simulink model "mlinear_SnookieConfiguration"  (R2017a)
settings: Solver=VariableStepAuto  StartTime=0.0  StopTime=10.0  RelTol=1e-3
undefined symbols (not defined in the file or in its folder): veh
libraries: sharedutil x6, sharedtransform x2, shared6dofsys x2
settings Model: Creator=yongyu  LastModifiedBy=yongyu

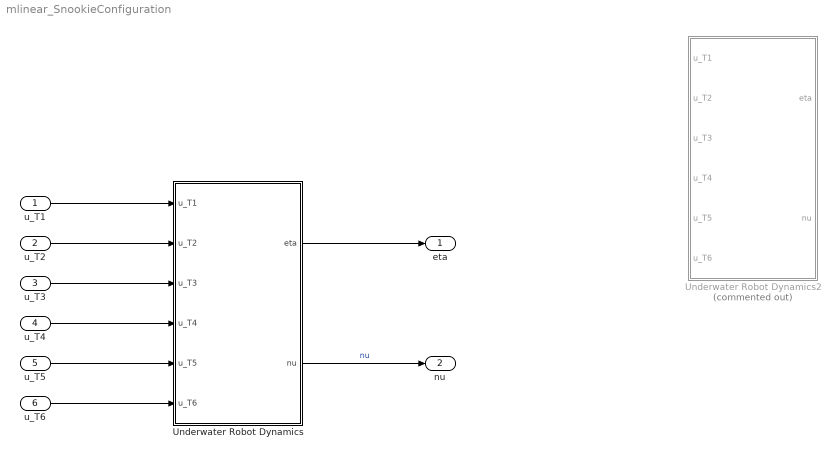
== system mlinear_SnookieConfiguration ==
  u_T1 : Inport
  u_T2 : Inport  Port=2
  u_T3 : Inport  Port=3
  u_T4 : Inport  Port=4
  u_T5 : Inport  Port=5
  u_T6 : Inport  Port=6
  Underwater Robot Dynamics : Subsystem
  Underwater Robot Dynamics2 : Subsystem  Commented=on
  eta : Outport
  nu : Outport  Port=2
  wires:
  u_T1/1 -> Underwater Robot Dynamics/1(u_T1)
  Underwater Robot Dynamics/1(eta) -> eta/1
  Underwater Robot Dynamics/2(nu) -> nu/1  "nu"
  u_T2/1 -> Underwater Robot Dynamics/2(u_T2)
  u_T3/1 -> Underwater Robot Dynamics/3(u_T3)
  u_T4/1 -> Underwater Robot Dynamics/4(u_T4)
  u_T5/1 -> Underwater Robot Dynamics/5(u_T5)
  u_T6/1 -> Underwater Robot Dynamics/6(u_T6)

== system mlinear_SnookieConfiguration/Underwater Robot Dynamics ==
  u_T1 : Inport
  u_T2 : Inport  Port=2
  u_T3 : Inport  Port=3
  u_T4 : Inport  Port=4
  u_T5 : Inport  Port=5
  u_T6 : Inport  Port=6
  ForceMomentTransfer : Subsystem
  Mux : Mux  Inputs=2
  Mux1 : Mux  Inputs=2
  Position Integrator(x,y,z) : Integrator
  Subsystem : Subsystem
  Transpose : Math  Operator=transpose  SaturateOnIntegerOverflow=on
  "Underwater Robot Dynamics " : Subsystem
  "transform to inertial world frame {i}" : Subsystem
  eta : Outport
  nu : Outport  Port=2
  wires:
  Transpose/1 -> "transform to inertial world frame {i}"/2(linear velocity transformation matrix)
  Mux1/1 -> nu/1  "nu"
  Mux/1 -> eta/1
  "transform to inertial world frame {i}"/1(Ve) -> Position Integrator(x,y,z)/1
  Position Integrator(x,y,z)/1 -> Mux/1
  "Underwater Robot Dynamics "/2(w_ib) -> Subsystem/1("p q r "), Mux1/2
  "Underwater Robot Dynamics "/1(v) -> Mux1/1, "transform to inertial world frame {i}"/1(v)
  Subsystem/1(DCM) -> Transpose/1
  Subsystem/2(Euler) -> Mux/2
  u_T1/1 -> ForceMomentTransfer/1(u_T1)
  u_T2/1 -> ForceMomentTransfer/2(u_T2)
  u_T3/1 -> ForceMomentTransfer/3(u_T3)
  u_T4/1 -> ForceMomentTransfer/4(u_T4)
  u_T5/1 -> ForceMomentTransfer/5(u_T5)
  u_T6/1 -> ForceMomentTransfer/6(u_T6)
  ForceMomentTransfer/1(tau_b) -> "Underwater Robot Dynamics "/1(tau_b)

== system mlinear_SnookieConfiguration/Underwater Robot Dynamics2 ==
  u_T1 : Inport
  u_T2 : Inport  Port=2
  u_T3 : Inport  Port=3
  u_T4 : Inport  Port=4
  u_T5 : Inport  Port=5
  u_T6 : Inport  Port=6
  ForceMomentTransfer : Subsystem
  Mux : Mux  Inputs=2
  Mux1 : Mux  Inputs=2
  Position Integrator(x,y,z) : Integrator
  Subsystem : Subsystem
  Transpose : Math  Operator=transpose  SaturateOnIntegerOverflow=on
  "Underwater Robot Dynamics " : Subsystem
  "transform to inertial world frame {i}" : Subsystem
  eta : Outport
  nu : Outport  Port=2
  wires:
  Transpose/1 -> "transform to inertial world frame {i}"/2(linear velocity transformation matrix)
  Mux1/1 -> nu/1  "nu"
  Mux/1 -> eta/1
  "transform to inertial world frame {i}"/1(Ve) -> Position Integrator(x,y,z)/1
  Position Integrator(x,y,z)/1 -> Mux/1
  "Underwater Robot Dynamics "/2(w_ib) -> Subsystem/1("p q r "), Mux1/2
  "Underwater Robot Dynamics "/1(v) -> Mux1/1, "transform to inertial world frame {i}"/1(v)
  Subsystem/1(DCM) -> Transpose/1
  Subsystem/2(Euler) -> Mux/2
  u_T1/1 -> ForceMomentTransfer/1(u_T1)
  u_T2/1 -> ForceMomentTransfer/2(u_T2)
  u_T3/1 -> ForceMomentTransfer/3(u_T3)
  u_T4/1 -> ForceMomentTransfer/4(u_T4)
  u_T5/1 -> ForceMomentTransfer/5(u_T5)
  u_T6/1 -> ForceMomentTransfer/6(u_T6)
  ForceMomentTransfer/1(tau_b) -> "Underwater Robot Dynamics "/1(tau_b)

== system mlinear_SnookieConfiguration/Underwater Robot Dynamics/ForceMomentTransfer ==
  u_T1 : Inport
  u_T2 : Inport  Port=2
  u_T3 : Inport  Port=3
  u_T4 : Inport  Port=4
  u_T5 : Inport  Port=5
  u_T6 : Inport  Port=6
  Mux : Mux  Inputs=2
  Total Force : Subsystem
  Total Moment : Subsystem
  tau_b : Outport
  wires:
  u_T1/1 -> Total Moment/1(u_T1), Total Force/1(u_T1)
  u_T2/1 -> Total Moment/2(u_T2), Total Force/2(u_T2)
  u_T3/1 -> Total Force/3(u_T3), Total Moment/3(u_T3)
  u_T4/1 -> Total Force/4(u_T4), Total Moment/4(u_T4)
  u_T5/1 -> Total Force/5(u_T5), Total Moment/5(u_T5)
  u_T6/1 -> Total Force/6(u_T6), Total Moment/6(u_T6)
  Total Force/1(F_T) -> Mux/1
  Total Moment/1(m_T) -> Mux/2
  Mux/1 -> tau_b/1

== system mlinear_SnookieConfiguration/Underwater Robot Dynamics/Subsystem ==
  "p q r " : Inport
  Rotation Angles to Direction Cosine Matrix : sharedtransform/Rotation Angles to Direction Cosine Matrix  rotationOrder=ZYX
  Selector : Selector  InputPortWidth=3  IndexOptions=Index vector (dialog)  Indices=[3 2 1]  OutputSizes=1
  phi theta psi : Integrator
  phidot thetadot psidot : shared6dofsys/DCM & Euler Angles (Euler)/phidot thetadot psidot
  DCM : Outport
  Euler : Outport  Port=2
  wires:
  Selector/1 -> Rotation Angles to Direction Cosine Matrix/1
  "p q r "/1 -> phidot thetadot psidot/1
  phi theta psi/1 -> Euler/1, Selector/1, phidot thetadot psidot/2
  phidot thetadot psidot/1 -> phi theta psi/1
  Rotation Angles to Direction Cosine Matrix/1 -> DCM/1

== system mlinear_SnookieConfiguration/Underwater Robot Dynamics/Underwater Robot Dynamics  ==
  tau_b : Inport
  6DOF Coriolis forces : Subsystem
  M_A : Constant  Value=veh.Ma
  M_RB : Constant  Value=veh.Mrb
  Product : Product  Inputs=/*  Multiplication=Matrix(*)  SaturateOnIntegerOverflow=on  OutDataTypeStr=Inherit: Same as first input
  Scope : Scope
  Selector1 : Selector  InputPortWidth=6  IndexOptions=Index vector (dialog)  Indices=[1 2 3]  OutputSizes=1
  Selector2 : Selector  InputPortWidth=6  IndexOptions=Index vector (dialog)  Indices=[4 5 6]  OutputSizes=1
  Sum : Sum  Inputs=|+-
  Sum2 : Sum  SaturateOnIntegerOverflow=on
  Velocity Integrator : Integrator
  v : Outport
  w_ib : Outport  Port=2
  wires:
  M_RB/1 -> Sum2/1
  M_A/1 -> Sum2/2
  Sum2/1 -> Product/1, 6DOF Coriolis forces/1(M)  "M"
  Selector2/1 -> w_ib/1  "w_nb"
  Product/1 -> Velocity Integrator/1  "(d/dt)nu"
  6DOF Coriolis forces/1(C(nu)nu) -> Sum/2, Scope/1
  Sum/1 -> Product/2
  Selector1/1 -> v/1  "v"
  Velocity Integrator/1 -> 6DOF Coriolis forces/2(nu), Selector2/1, Selector1/1  "nu"
  tau_b/1 -> Sum/1

== system mlinear_SnookieConfiguration/Underwater Robot Dynamics/transform to inertial world frame {i} ==
  v : Inport
  linear velocity transformation matrix : Inport  Port=2
  Product : Product  Multiplication=Matrix(*)  SaturateOnIntegerOverflow=on  InputSameDT=on  OutDataTypeStr=Inherit: Same as first input
  Reshape1 : Reshape  OutputDimensionality=Column vector (2-D)
  Reshape2 : Reshape
  Ve : Outport
  wires:
  Product/1 -> Reshape2/1
  Reshape1/1 -> Product/2
  v/1 -> Reshape1/1
  Reshape2/1 -> Ve/1
  linear velocity transformation matrix/1 -> Product/1

== system mlinear_SnookieConfiguration/Underwater Robot Dynamics2/ForceMomentTransfer ==
  u_T1 : Inport
  u_T2 : Inport  Port=2
  u_T3 : Inport  Port=3
  u_T4 : Inport  Port=4
  u_T5 : Inport  Port=5
  u_T6 : Inport  Port=6
  Mux : Mux  Inputs=2
  Total Force : Subsystem
  Total Moment : Subsystem
  tau_b : Outport
  wires:
  u_T1/1 -> Total Moment/1(u_T1), Total Force/1(u_T1)
  u_T2/1 -> Total Moment/2(u_T2), Total Force/2(u_T2)
  u_T3/1 -> Total Force/3(u_T3), Total Moment/3(u_T3)
  u_T4/1 -> Total Force/4(u_T4), Total Moment/4(u_T4)
  u_T5/1 -> Total Force/5(u_T5), Total Moment/5(u_T5)
  u_T6/1 -> Total Force/6(u_T6), Total Moment/6(u_T6)
  Total Force/1(F_T) -> Mux/1
  Total Moment/1(m_T) -> Mux/2
  Mux/1 -> tau_b/1

== system mlinear_SnookieConfiguration/Underwater Robot Dynamics2/Subsystem ==
  "p q r " : Inport
  Rotation Angles to Direction Cosine Matrix : sharedtransform/Rotation Angles to Direction Cosine Matrix  rotationOrder=ZYX
  Selector : Selector  InputPortWidth=3  IndexOptions=Index vector (dialog)  Indices=[3 2 1]  OutputSizes=1
  phi theta psi : Integrator
  phidot thetadot psidot : shared6dofsys/DCM & Euler Angles (Euler)/phidot thetadot psidot
  DCM : Outport
  Euler : Outport  Port=2
  wires:
  Selector/1 -> Rotation Angles to Direction Cosine Matrix/1
  "p q r "/1 -> phidot thetadot psidot/1
  phi theta psi/1 -> Euler/1, Selector/1, phidot thetadot psidot/2
  phidot thetadot psidot/1 -> phi theta psi/1
  Rotation Angles to Direction Cosine Matrix/1 -> DCM/1

== system mlinear_SnookieConfiguration/Underwater Robot Dynamics2/Underwater Robot Dynamics  ==
  tau_b : Inport
  6DOF Coriolis forces : Subsystem
  M_A : Constant  Value=veh.Ma
  M_RB : Constant  Value=veh.Mrb
  Product : Product  Inputs=/*  Multiplication=Matrix(*)  SaturateOnIntegerOverflow=on  OutDataTypeStr=Inherit: Same as first input
  Scope : Scope
  Selector1 : Selector  InputPortWidth=6  IndexOptions=Index vector (dialog)  Indices=[1 2 3]  OutputSizes=1
  Selector2 : Selector  InputPortWidth=6  IndexOptions=Index vector (dialog)  Indices=[4 5 6]  OutputSizes=1
  Sum : Sum  Inputs=|+-
  Sum2 : Sum  SaturateOnIntegerOverflow=on
  Velocity Integrator : Integrator
  v : Outport
  w_ib : Outport  Port=2
  wires:
  M_RB/1 -> Sum2/1
  M_A/1 -> Sum2/2
  Sum2/1 -> Product/1, 6DOF Coriolis forces/1(M)  "M"
  Selector2/1 -> w_ib/1  "w_nb"
  Product/1 -> Velocity Integrator/1  "(d/dt)nu"
  6DOF Coriolis forces/1(C(nu)nu) -> Sum/2, Scope/1
  Sum/1 -> Product/2
  Selector1/1 -> v/1  "v"
  Velocity Integrator/1 -> 6DOF Coriolis forces/2(nu), Selector2/1, Selector1/1  "nu"
  tau_b/1 -> Sum/1

== system mlinear_SnookieConfiguration/Underwater Robot Dynamics2/transform to inertial world frame {i} ==
  v : Inport
  linear velocity transformation matrix : Inport  Port=2
  Product : Product  Multiplication=Matrix(*)  SaturateOnIntegerOverflow=on  InputSameDT=on  OutDataTypeStr=Inherit: Same as first input
  Reshape1 : Reshape  OutputDimensionality=Column vector (2-D)
  Reshape2 : Reshape
  Ve : Outport
  wires:
  Product/1 -> Reshape2/1
  Reshape1/1 -> Product/2
  v/1 -> Reshape1/1
  Reshape2/1 -> Ve/1
  linear velocity transformation matrix/1 -> Product/1

== system mlinear_SnookieConfiguration/Underwater Robot Dynamics/ForceMomentTransfer/Total Force ==
  u_T1 : Inport
  u_T2 : Inport  Port=2
  u_T3 : Inport  Port=3
  u_T4 : Inport  Port=4
  u_T5 : Inport  Port=5
  u_T6 : Inport  Port=6
  Add : Sum  Inputs=++++++
  Gain : Gain  Gain=veh.d_T1
  Gain1 : Gain  Gain=veh.d_T2
  Gain2 : Gain  Gain=veh.d_T3
  Gain3 : Gain  Gain=veh.d_T4
  Gain4 : Gain  Gain=veh.d_T5
  Gain5 : Gain  Gain=veh.d_T6
  F_T : Outport
  wires:
  Add/1 -> F_T/1
  u_T1/1 -> Gain/1
  Gain/1 -> Add/1
  Gain1/1 -> Add/2
  Gain2/1 -> Add/3
  u_T2/1 -> Gain1/1
  u_T3/1 -> Gain2/1
  Gain3/1 -> Add/4
  u_T4/1 -> Gain3/1
  u_T5/1 -> Gain4/1
  Gain4/1 -> Add/5
  u_T6/1 -> Gain5/1
  Gain5/1 -> Add/6

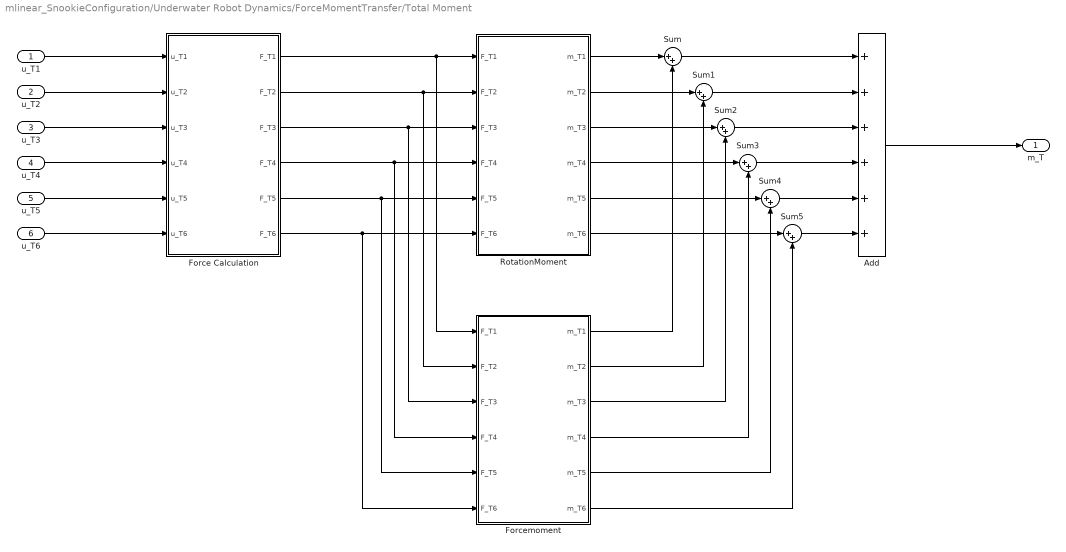
== system mlinear_SnookieConfiguration/Underwater Robot Dynamics/ForceMomentTransfer/Total Moment ==
  u_T1 : Inport
  u_T2 : Inport  Port=2
  u_T3 : Inport  Port=3
  u_T4 : Inport  Port=4
  u_T5 : Inport  Port=5
  u_T6 : Inport  Port=6
  Add : Sum  Inputs=++++++
  "Force Calculation " : Subsystem
  Forcemoment : Subsystem
  RotationMoment : Subsystem
  Sum{,1..5} (6 alike) : Sum  Inputs=|++
  m_T : Outport
  wires:
  Add/1 -> m_T/1
  "Force Calculation "/1(F_T1) -> Forcemoment/1(F_T1), RotationMoment/1(F_T1)
  "Force Calculation "/2(F_T2) -> Forcemoment/2(F_T2), RotationMoment/2(F_T2)
  "Force Calculation "/3(F_T3) -> Forcemoment/3(F_T3), RotationMoment/3(F_T3)
  "Force Calculation "/5(F_T5) -> Forcemoment/5(F_T5), RotationMoment/5(F_T5)
  "Force Calculation "/4(F_T4) -> Forcemoment/4(F_T4), RotationMoment/4(F_T4)
  "Force Calculation "/6(F_T6) -> Forcemoment/6(F_T6), RotationMoment/6(F_T6)
  RotationMoment/1(m_T1) -> Sum/1
  Forcemoment/1(m_T1) -> Sum/2
  RotationMoment/2(m_T2) -> Sum1/1
  Forcemoment/2(m_T2) -> Sum1/2
  RotationMoment/3(m_T3) -> Sum2/1
  Forcemoment/3(m_T3) -> Sum2/2
  RotationMoment/4(m_T4) -> Sum3/1
  Forcemoment/4(m_T4) -> Sum3/2
  RotationMoment/5(m_T5) -> Sum4/1
  Forcemoment/5(m_T5) -> Sum4/2
  RotationMoment/6(m_T6) -> Sum5/1
  Forcemoment/6(m_T6) -> Sum5/2
  Sum/1 -> Add/1
  Sum1/1 -> Add/2
  Sum2/1 -> Add/3
  Sum3/1 -> Add/4
  Sum4/1 -> Add/5
  Sum5/1 -> Add/6
  u_T1/1 -> "Force Calculation "/1(u_T1)
  u_T2/1 -> "Force Calculation "/2(u_T2)
  u_T3/1 -> "Force Calculation "/3(u_T3)
  u_T4/1 -> "Force Calculation "/4(u_T4)
  u_T5/1 -> "Force Calculation "/5(u_T5)
  u_T6/1 -> "Force Calculation "/6(u_T6)

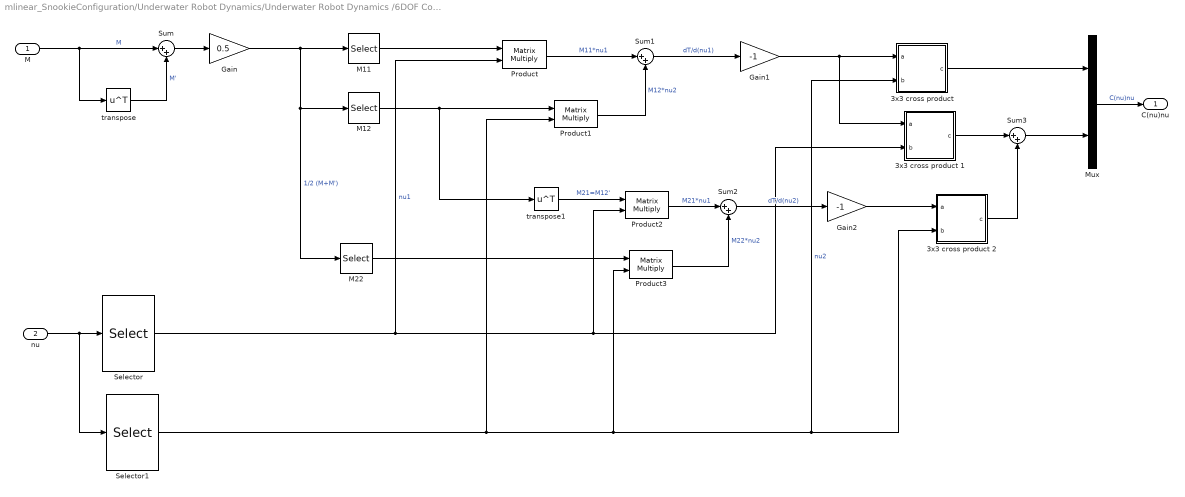
== system mlinear_SnookieConfiguration/Underwater Robot Dynamics/Underwater Robot Dynamics /6DOF Coriolis forces ==
  M : Inport
  nu : Inport  Port=2
  3x3 cross product : Subsystem
  3x3 cross product 1 : Subsystem
  3x3 cross product 2 : Subsystem
  Gain : Gain  Gain=0.5  SaturateOnIntegerOverflow=on  OutDataTypeStr=Inherit: Same as input  ParamDataTypeStr=Inherit: Same as input
  Gain1 : Gain  Gain=-1  SaturateOnIntegerOverflow=on  OutDataTypeStr=Inherit: Same as input  ParamDataTypeStr=Inherit: Same as input
  Gain2 : Gain  Gain=-1  SaturateOnIntegerOverflow=on  OutDataTypeStr=Inherit: Same as input  ParamDataTypeStr=Inherit: Same as input
  M11 : Selector  NumberOfDimensions=2  InputPortWidth=3  IndexOptions=Index vector (dialog),Index vector (dialog)  Indices=[1 2 3],[1 2 3]  OutputSizes=1
  M12 : Selector  NumberOfDimensions=2  InputPortWidth=3  IndexOptions=Index vector (dialog),Index vector (dialog)  Indices=[1 2 3],[4 5 6]  OutputSizes=1
  M22 : Selector  NumberOfDimensions=2  InputPortWidth=3  IndexOptions=Index vector (dialog),Index vector (dialog)  Indices=[4 5 6],[4 5 6]  OutputSizes=1
  Mux : Mux  Inputs=2
  Product{,1..3} (4 alike) : Product  Multiplication=Matrix(*)  SaturateOnIntegerOverflow=on  OutDataTypeStr=Inherit: Same as first input
  Selector : Selector  InputPortWidth=6  IndexOptions=Index vector (dialog)  Indices=[1 2 3]  OutputSizes=1
  Selector1 : Selector  InputPortWidth=6  IndexOptions=Index vector (dialog)  Indices=[4 5 6]  OutputSizes=1
  Sum{,1..3} (4 alike) : Sum  Inputs=|++  SaturateOnIntegerOverflow=on
  transpose : Math  Operator=transpose  SaturateOnIntegerOverflow=on
  transpose1 : Math  Operator=transpose  SaturateOnIntegerOverflow=on
  C(nu)nu : Outport
  wires:
  transpose/1 -> Sum/2  "M'"
  Sum/1 -> Gain/1
  Gain/1 -> M22/1, M12/1, M11/1  "1/2 (M+M')"
  Selector/1 -> Product2/2, 3x3 cross product 1/2(b), Product/2  "nu1"
  Selector1/1 -> 3x3 cross product/2(b), 3x3 cross product 2/2(b), Product3/2, Product1/2  "nu2"
  M11/1 -> Product/1
  Product/1 -> Sum1/1  "M11*nu1"
  M12/1 -> transpose1/1, Product1/1
  Product1/1 -> Sum1/2  "M12*nu2"
  Sum1/1 -> Gain1/1  "dT/d(nu1)"
  transpose1/1 -> Product2/1  "M21=M12'"
  Product2/1 -> Sum2/1  "M21*nu1"
  M22/1 -> Product3/1
  Product3/1 -> Sum2/2  "M22*nu2"
  Sum2/1 -> Gain2/1  "dT/d(nu2)"
  Gain1/1 -> 3x3 cross product/1(a), 3x3 cross product 1/1(a)
  3x3 cross product/1(c) -> Mux/1
  Gain2/1 -> 3x3 cross product 2/1(a)
  3x3 cross product 1/1(c) -> Sum3/1
  3x3 cross product 2/1(c) -> Sum3/2
  Sum3/1 -> Mux/2
  Mux/1 -> C(nu)nu/1  "C(nu)nu"
  nu/1 -> Selector/1, Selector1/1
  M/1 -> transpose/1, Sum/1  "M"

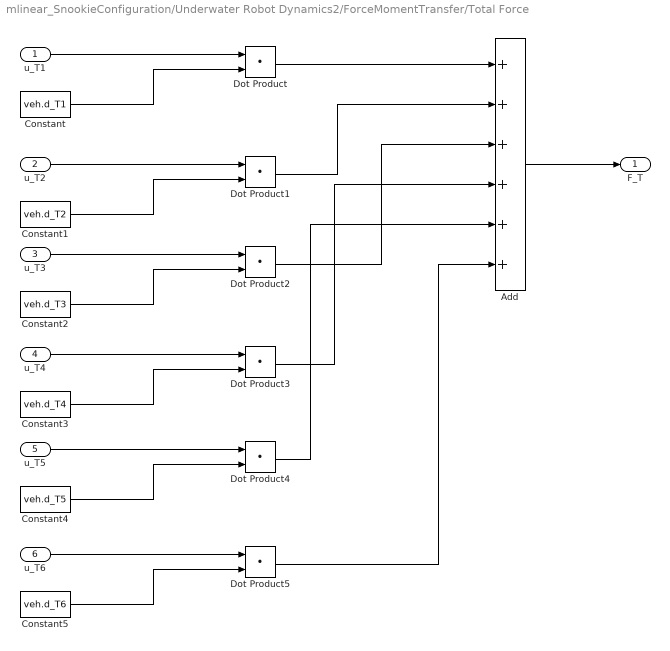
== system mlinear_SnookieConfiguration/Underwater Robot Dynamics2/ForceMomentTransfer/Total Force ==
  u_T1 : Inport
  u_T2 : Inport  Port=2
  u_T3 : Inport  Port=3
  u_T4 : Inport  Port=4
  u_T5 : Inport  Port=5
  u_T6 : Inport  Port=6
  Add : Sum  Inputs=++++++
  Constant : Constant  Value=veh.d_T1
  Constant1 : Constant  Value=veh.d_T2
  Constant2 : Constant  Value=veh.d_T3
  Constant3 : Constant  Value=veh.d_T4
  Constant4 : Constant  Value=veh.d_T5
  Constant5 : Constant  Value=veh.d_T6
  Dot Product{,1..5} (6 alike) : DotProduct  InputSameDT=on  OutDataTypeStr=Inherit: Inherit via internal rule
  F_T : Outport
  wires:
  Add/1 -> F_T/1
  u_T1/1 -> Dot Product/1
  Constant/1 -> Dot Product/2
  Dot Product/1 -> Add/1
  Constant1/1 -> Dot Product1/2
  u_T2/1 -> Dot Product1/1
  Dot Product1/1 -> Add/2
  u_T3/1 -> Dot Product2/1
  Constant2/1 -> Dot Product2/2
  Dot Product2/1 -> Add/3
  u_T4/1 -> Dot Product3/1
  Constant3/1 -> Dot Product3/2
  Dot Product3/1 -> Add/4
  u_T5/1 -> Dot Product4/1
  Constant4/1 -> Dot Product4/2
  u_T6/1 -> Dot Product5/1
  Constant5/1 -> Dot Product5/2
  Dot Product4/1 -> Add/5
  Dot Product5/1 -> Add/6

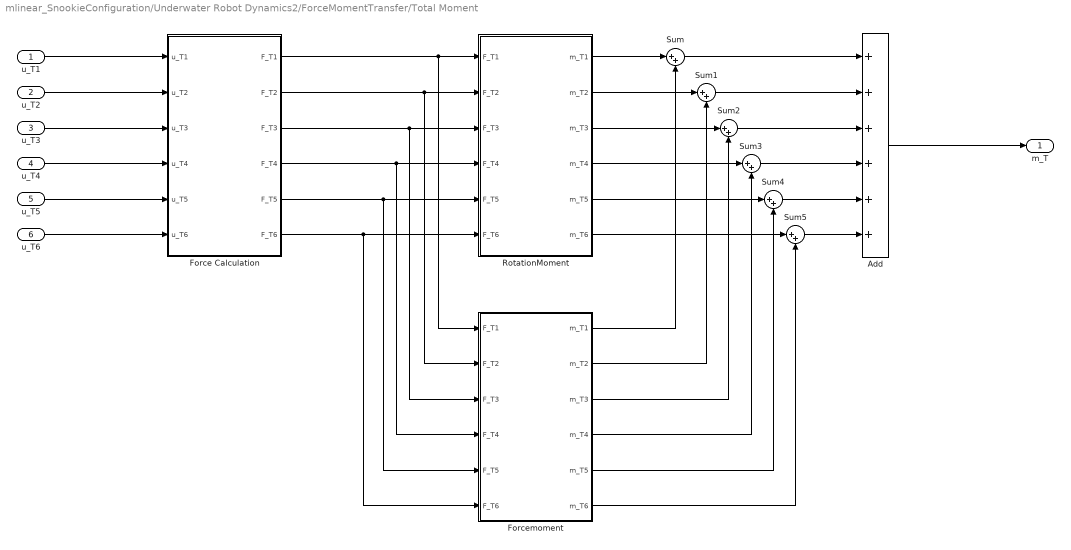
== system mlinear_SnookieConfiguration/Underwater Robot Dynamics2/ForceMomentTransfer/Total Moment ==
  u_T1 : Inport
  u_T2 : Inport  Port=2
  u_T3 : Inport  Port=3
  u_T4 : Inport  Port=4
  u_T5 : Inport  Port=5
  u_T6 : Inport  Port=6
  Add : Sum  Inputs=++++++
  "Force Calculation " : Subsystem
  Forcemoment : Subsystem
  RotationMoment : Subsystem
  Sum{,1..5} (6 alike) : Sum  Inputs=|++
  m_T : Outport
  wires:
  Add/1 -> m_T/1
  u_T1/1 -> "Force Calculation "/1(u_T1)
  u_T3/1 -> "Force Calculation "/3(u_T3)
  u_T4/1 -> "Force Calculation "/4(u_T4)
  u_T2/1 -> "Force Calculation "/2(u_T2)
  u_T5/1 -> "Force Calculation "/5(u_T5)
  u_T6/1 -> "Force Calculation "/6(u_T6)
  "Force Calculation "/1(F_T1) -> Forcemoment/1(F_T1), RotationMoment/1(F_T1)
  "Force Calculation "/2(F_T2) -> Forcemoment/2(F_T2), RotationMoment/2(F_T2)
  "Force Calculation "/3(F_T3) -> Forcemoment/3(F_T3), RotationMoment/3(F_T3)
  "Force Calculation "/5(F_T5) -> Forcemoment/5(F_T5), RotationMoment/5(F_T5)
  "Force Calculation "/4(F_T4) -> Forcemoment/4(F_T4), RotationMoment/4(F_T4)
  "Force Calculation "/6(F_T6) -> Forcemoment/6(F_T6), RotationMoment/6(F_T6)
  RotationMoment/1(m_T1) -> Sum/1
  Forcemoment/1(m_T1) -> Sum/2
  RotationMoment/2(m_T2) -> Sum1/1
  Forcemoment/2(m_T2) -> Sum1/2
  RotationMoment/3(m_T3) -> Sum2/1
  Forcemoment/3(m_T3) -> Sum2/2
  RotationMoment/4(m_T4) -> Sum3/1
  Forcemoment/4(m_T4) -> Sum3/2
  RotationMoment/5(m_T5) -> Sum4/1
  Forcemoment/5(m_T5) -> Sum4/2
  RotationMoment/6(m_T6) -> Sum5/1
  Forcemoment/6(m_T6) -> Sum5/2
  Sum/1 -> Add/1
  Sum1/1 -> Add/2
  Sum2/1 -> Add/3
  Sum3/1 -> Add/4
  Sum4/1 -> Add/5
  Sum5/1 -> Add/6

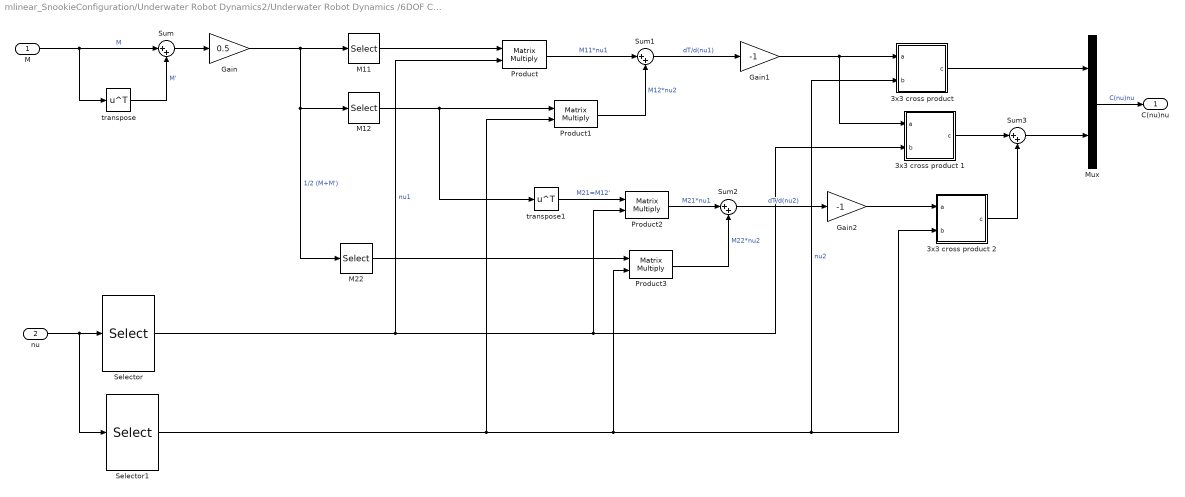
== system mlinear_SnookieConfiguration/Underwater Robot Dynamics2/Underwater Robot Dynamics /6DOF Coriolis forces ==
  M : Inport
  nu : Inport  Port=2
  3x3 cross product : Subsystem
  3x3 cross product 1 : Subsystem
  3x3 cross product 2 : Subsystem
  Gain : Gain  Gain=0.5  SaturateOnIntegerOverflow=on  OutDataTypeStr=Inherit: Same as input  ParamDataTypeStr=Inherit: Same as input
  Gain1 : Gain  Gain=-1  SaturateOnIntegerOverflow=on  OutDataTypeStr=Inherit: Same as input  ParamDataTypeStr=Inherit: Same as input
  Gain2 : Gain  Gain=-1  SaturateOnIntegerOverflow=on  OutDataTypeStr=Inherit: Same as input  ParamDataTypeStr=Inherit: Same as input
  M11 : Selector  NumberOfDimensions=2  InputPortWidth=3  IndexOptions=Index vector (dialog),Index vector (dialog)  Indices=[1 2 3],[1 2 3]  OutputSizes=1
  M12 : Selector  NumberOfDimensions=2  InputPortWidth=3  IndexOptions=Index vector (dialog),Index vector (dialog)  Indices=[1 2 3],[4 5 6]  OutputSizes=1
  M22 : Selector  NumberOfDimensions=2  InputPortWidth=3  IndexOptions=Index vector (dialog),Index vector (dialog)  Indices=[4 5 6],[4 5 6]  OutputSizes=1
  Mux : Mux  Inputs=2
  Product{,1..3} (4 alike) : Product  Multiplication=Matrix(*)  SaturateOnIntegerOverflow=on  OutDataTypeStr=Inherit: Same as first input
  Selector : Selector  InputPortWidth=6  IndexOptions=Index vector (dialog)  Indices=[1 2 3]  OutputSizes=1
  Selector1 : Selector  InputPortWidth=6  IndexOptions=Index vector (dialog)  Indices=[4 5 6]  OutputSizes=1
  Sum{,1..3} (4 alike) : Sum  Inputs=|++  SaturateOnIntegerOverflow=on
  transpose : Math  Operator=transpose  SaturateOnIntegerOverflow=on
  transpose1 : Math  Operator=transpose  SaturateOnIntegerOverflow=on
  C(nu)nu : Outport
  wires:
  transpose/1 -> Sum/2  "M'"
  Sum/1 -> Gain/1
  Gain/1 -> M22/1, M12/1, M11/1  "1/2 (M+M')"
  Selector/1 -> Product2/2, 3x3 cross product 1/2(b), Product/2  "nu1"
  Selector1/1 -> 3x3 cross product/2(b), 3x3 cross product 2/2(b), Product3/2, Product1/2  "nu2"
  M11/1 -> Product/1
  Product/1 -> Sum1/1  "M11*nu1"
  M12/1 -> transpose1/1, Product1/1
  Product1/1 -> Sum1/2  "M12*nu2"
  Sum1/1 -> Gain1/1  "dT/d(nu1)"
  transpose1/1 -> Product2/1  "M21=M12'"
  Product2/1 -> Sum2/1  "M21*nu1"
  M22/1 -> Product3/1
  Product3/1 -> Sum2/2  "M22*nu2"
  Sum2/1 -> Gain2/1  "dT/d(nu2)"
  Gain1/1 -> 3x3 cross product/1(a), 3x3 cross product 1/1(a)
  3x3 cross product/1(c) -> Mux/1
  Gain2/1 -> 3x3 cross product 2/1(a)
  3x3 cross product 1/1(c) -> Sum3/1
  3x3 cross product 2/1(c) -> Sum3/2
  Sum3/1 -> Mux/2
  Mux/1 -> C(nu)nu/1  "C(nu)nu"
  nu/1 -> Selector/1, Selector1/1
  M/1 -> transpose/1, Sum/1  "M"

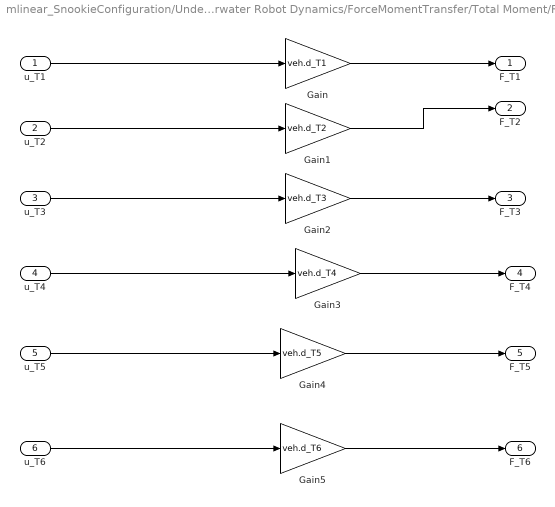
== system mlinear_SnookieConfiguration/Underwater Robot Dynamics/ForceMomentTransfer/Total Moment/Force Calculation  ==
  u_T1 : Inport
  u_T2 : Inport  Port=2
  u_T3 : Inport  Port=3
  u_T4 : Inport  Port=4
  u_T5 : Inport  Port=5
  u_T6 : Inport  Port=6
  Gain : Gain  Gain=veh.d_T1
  Gain1 : Gain  Gain=veh.d_T2
  Gain2 : Gain  Gain=veh.d_T3
  Gain3 : Gain  Gain=veh.d_T4
  Gain4 : Gain  Gain=veh.d_T5
  Gain5 : Gain  Gain=veh.d_T6
  F_T1 : Outport
  F_T2 : Outport  Port=2
  F_T3 : Outport  Port=3
  F_T4 : Outport  Port=4
  F_T5 : Outport  Port=5
  F_T6 : Outport  Port=6
  wires:
  u_T3/1 -> Gain2/1
  u_T6/1 -> Gain5/1
  u_T2/1 -> Gain1/1
  u_T4/1 -> Gain3/1
  Gain/1 -> F_T1/1
  u_T1/1 -> Gain/1
  u_T5/1 -> Gain4/1
  Gain1/1 -> F_T2/1
  Gain2/1 -> F_T3/1
  Gain3/1 -> F_T4/1
  Gain4/1 -> F_T5/1
  Gain5/1 -> F_T6/1

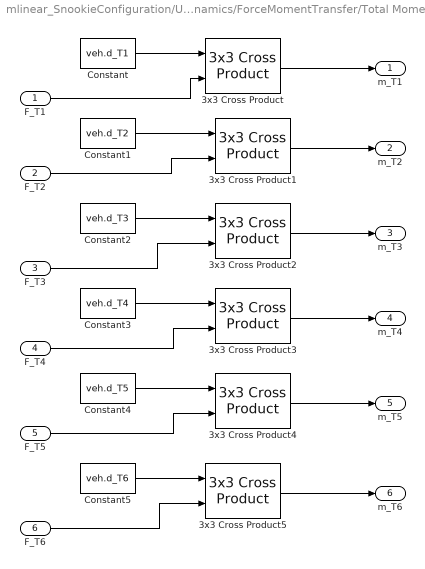
== system mlinear_SnookieConfiguration/Underwater Robot Dynamics/ForceMomentTransfer/Total Moment/Forcemoment ==
  F_T1 : Inport
  F_T2 : Inport  Port=2
  F_T3 : Inport  Port=3
  F_T4 : Inport  Port=4
  F_T5 : Inport  Port=5
  F_T6 : Inport  Port=6
  3x3 Cross Product{,1..5} (6 alike) : sharedutil/3x3 Cross Product
  Constant : Constant  Value=veh.d_T1
  Constant1 : Constant  Value=veh.d_T2
  Constant2 : Constant  Value=veh.d_T3
  Constant3 : Constant  Value=veh.d_T4
  Constant4 : Constant  Value=veh.d_T5
  Constant5 : Constant  Value=veh.d_T6
  m_T1 : Outport
  m_T2 : Outport  Port=2
  m_T3 : Outport  Port=3
  m_T4 : Outport  Port=4
  m_T5 : Outport  Port=5
  m_T6 : Outport  Port=6
  wires:
  F_T2/1 -> 3x3 Cross Product1/2
  F_T6/1 -> 3x3 Cross Product5/2
  F_T4/1 -> 3x3 Cross Product3/2
  Constant/1 -> 3x3 Cross Product/1
  Constant1/1 -> 3x3 Cross Product1/1
  Constant2/1 -> 3x3 Cross Product2/1
  F_T3/1 -> 3x3 Cross Product2/2
  Constant3/1 -> 3x3 Cross Product3/1
  Constant4/1 -> 3x3 Cross Product4/1
  F_T5/1 -> 3x3 Cross Product4/2
  Constant5/1 -> 3x3 Cross Product5/1
  3x3 Cross Product/1 -> m_T1/1
  3x3 Cross Product1/1 -> m_T2/1
  3x3 Cross Product2/1 -> m_T3/1
  3x3 Cross Product3/1 -> m_T4/1
  3x3 Cross Product4/1 -> m_T5/1
  3x3 Cross Product5/1 -> m_T6/1
  F_T1/1 -> 3x3 Cross Product/2

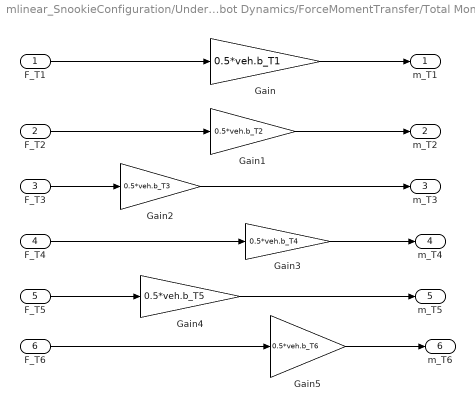
== system mlinear_SnookieConfiguration/Underwater Robot Dynamics/ForceMomentTransfer/Total Moment/RotationMoment ==
  F_T1 : Inport
  F_T2 : Inport  Port=2
  F_T3 : Inport  Port=3
  F_T4 : Inport  Port=4
  F_T5 : Inport  Port=5
  F_T6 : Inport  Port=6
  Gain : Gain  Gain=0.5*veh.b_T1
  Gain1 : Gain  Gain=0.5*veh.b_T2
  Gain2 : Gain  Gain=0.5*veh.b_T3
  Gain3 : Gain  Gain=0.5*veh.b_T4
  Gain4 : Gain  Gain=0.5*veh.b_T5
  Gain5 : Gain  Gain=0.5*veh.b_T6
  m_T1 : Outport
  m_T2 : Outport  Port=2
  m_T3 : Outport  Port=3
  m_T4 : Outport  Port=4
  m_T5 : Outport  Port=5
  m_T6 : Outport  Port=6
  wires:
  F_T1/1 -> Gain/1
  F_T3/1 -> Gain2/1
  Gain/1 -> m_T1/1
  F_T4/1 -> Gain3/1
  F_T6/1 -> Gain5/1
  F_T2/1 -> Gain1/1
  F_T5/1 -> Gain4/1
  Gain1/1 -> m_T2/1
  Gain2/1 -> m_T3/1
  Gain3/1 -> m_T4/1
  Gain4/1 -> m_T5/1
  Gain5/1 -> m_T6/1

== system mlinear_SnookieConfiguration/Underwater Robot Dynamics/Underwater Robot Dynamics /6DOF Coriolis forces/3x3 cross product ==
  a : Inport
  b : Inport  Port=2
  Product : Product  SaturateOnIntegerOverflow=on  InputSameDT=on  OutDataTypeStr=Inherit: Same as first input
  Product1 : Product  SaturateOnIntegerOverflow=on  InputSameDT=on  OutDataTypeStr=Inherit: Same as first input
  Selector : Selector  InputPortWidth=3  IndexOptions=Index vector (dialog)  Indices=[2 3 1]  OutputSizes=1
  Selector1 : Selector  InputPortWidth=3  IndexOptions=Index vector (dialog)  Indices=[3 1 2]  OutputSizes=1
  Selector2 : Selector  InputPortWidth=3  IndexOptions=Index vector (dialog)  Indices=[2 3 1]  OutputSizes=1
  Selector3 : Selector  InputPortWidth=3  IndexOptions=Index vector (dialog)  Indices=[3 1 2]  OutputSizes=1
  Sum : Sum  Inputs=+|-  SaturateOnIntegerOverflow=on  InputSameDT=on  OutDataTypeStr=Inherit: Same as first input
  c : Outport  InitialOutput=0
  wires:
  Selector3/1 -> Product1/1
  Selector2/1 -> Product1/2
  Product1/1 -> Sum/2
  Selector1/1 -> Product/2
  Product/1 -> Sum/1
  a/1 -> Selector3/1, Selector/1
  Selector/1 -> Product/1
  b/1 -> Selector2/1, Selector1/1
  Sum/1 -> c/1

== system mlinear_SnookieConfiguration/Underwater Robot Dynamics/Underwater Robot Dynamics /6DOF Coriolis forces/3x3 cross product 1 ==
  a : Inport
  b : Inport  Port=2
  Product : Product  SaturateOnIntegerOverflow=on  InputSameDT=on  OutDataTypeStr=Inherit: Same as first input
  Product1 : Product  SaturateOnIntegerOverflow=on  InputSameDT=on  OutDataTypeStr=Inherit: Same as first input
  Selector : Selector  InputPortWidth=3  IndexOptions=Index vector (dialog)  Indices=[2 3 1]  OutputSizes=1
  Selector1 : Selector  InputPortWidth=3  IndexOptions=Index vector (dialog)  Indices=[3 1 2]  OutputSizes=1
  Selector2 : Selector  InputPortWidth=3  IndexOptions=Index vector (dialog)  Indices=[2 3 1]  OutputSizes=1
  Selector3 : Selector  InputPortWidth=3  IndexOptions=Index vector (dialog)  Indices=[3 1 2]  OutputSizes=1
  Sum : Sum  Inputs=+|-  SaturateOnIntegerOverflow=on  InputSameDT=on  OutDataTypeStr=Inherit: Same as first input
  c : Outport  InitialOutput=0
  wires:
  Selector3/1 -> Product1/1
  Selector2/1 -> Product1/2
  Product1/1 -> Sum/2
  Selector1/1 -> Product/2
  Product/1 -> Sum/1
  a/1 -> Selector3/1, Selector/1
  Selector/1 -> Product/1
  b/1 -> Selector2/1, Selector1/1
  Sum/1 -> c/1

== system mlinear_SnookieConfiguration/Underwater Robot Dynamics/Underwater Robot Dynamics /6DOF Coriolis forces/3x3 cross product 2 ==
  a : Inport
  b : Inport  Port=2
  Product : Product  SaturateOnIntegerOverflow=on  InputSameDT=on  OutDataTypeStr=Inherit: Same as first input
  Product1 : Product  SaturateOnIntegerOverflow=on  InputSameDT=on  OutDataTypeStr=Inherit: Same as first input
  Selector : Selector  InputPortWidth=3  IndexOptions=Index vector (dialog)  Indices=[2 3 1]  OutputSizes=1
  Selector1 : Selector  InputPortWidth=3  IndexOptions=Index vector (dialog)  Indices=[3 1 2]  OutputSizes=1
  Selector2 : Selector  InputPortWidth=3  IndexOptions=Index vector (dialog)  Indices=[2 3 1]  OutputSizes=1
  Selector3 : Selector  InputPortWidth=3  IndexOptions=Index vector (dialog)  Indices=[3 1 2]  OutputSizes=1
  Sum : Sum  Inputs=+|-  SaturateOnIntegerOverflow=on  InputSameDT=on  OutDataTypeStr=Inherit: Same as first input
  c : Outport  InitialOutput=0
  wires:
  Selector3/1 -> Product1/1
  Selector2/1 -> Product1/2
  Product1/1 -> Sum/2
  Selector1/1 -> Product/2
  Product/1 -> Sum/1
  a/1 -> Selector3/1, Selector/1
  Selector/1 -> Product/1
  b/1 -> Selector2/1, Selector1/1
  Sum/1 -> c/1

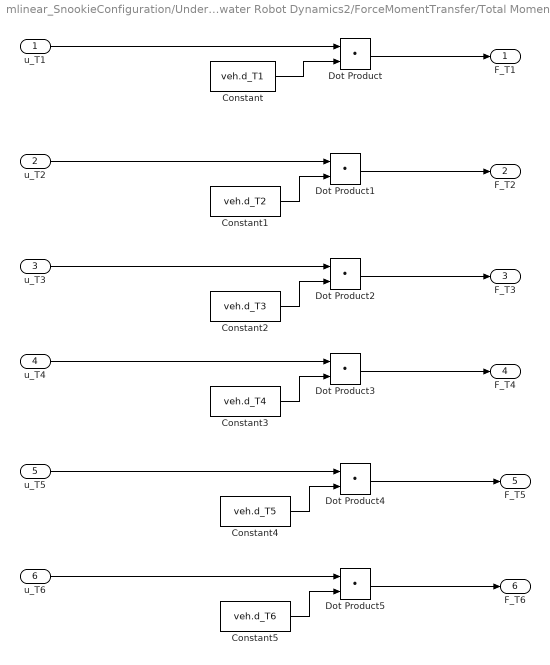
== system mlinear_SnookieConfiguration/Underwater Robot Dynamics2/ForceMomentTransfer/Total Moment/Force Calculation  ==
  u_T1 : Inport
  u_T2 : Inport  Port=2
  u_T3 : Inport  Port=3
  u_T4 : Inport  Port=4
  u_T5 : Inport  Port=5
  u_T6 : Inport  Port=6
  Constant : Constant  Value=veh.d_T1
  Constant1 : Constant  Value=veh.d_T2
  Constant2 : Constant  Value=veh.d_T3
  Constant3 : Constant  Value=veh.d_T4
  Constant4 : Constant  Value=veh.d_T5
  Constant5 : Constant  Value=veh.d_T6
  Dot Product{,1..5} (6 alike) : DotProduct  InputSameDT=on  OutDataTypeStr=Inherit: Inherit via internal rule
  F_T1 : Outport
  F_T2 : Outport  Port=2
  F_T3 : Outport  Port=3
  F_T4 : Outport  Port=4
  F_T5 : Outport  Port=5
  F_T6 : Outport  Port=6
  wires:
  u_T1/1 -> Dot Product/1
  Constant/1 -> Dot Product/2
  Constant1/1 -> Dot Product1/2
  u_T2/1 -> Dot Product1/1
  Dot Product/1 -> F_T1/1
  Dot Product1/1 -> F_T2/1
  Constant2/1 -> Dot Product2/2
  u_T3/1 -> Dot Product2/1
  Dot Product2/1 -> F_T3/1
  Constant3/1 -> Dot Product3/2
  u_T4/1 -> Dot Product3/1
  Dot Product3/1 -> F_T4/1
  Dot Product4/1 -> F_T5/1
  Constant4/1 -> Dot Product4/2
  u_T5/1 -> Dot Product4/1
  Constant5/1 -> Dot Product5/2
  u_T6/1 -> Dot Product5/1
  Dot Product5/1 -> F_T6/1

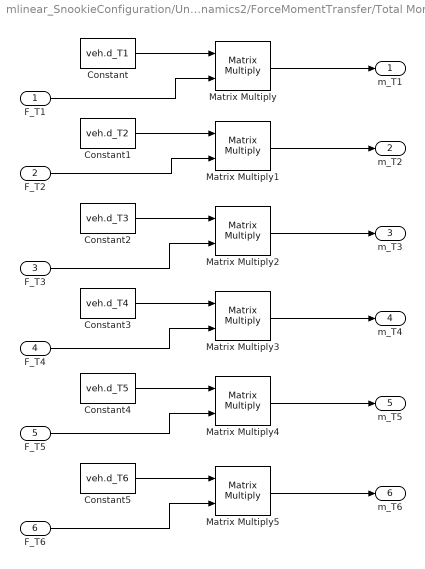
== system mlinear_SnookieConfiguration/Underwater Robot Dynamics2/ForceMomentTransfer/Total Moment/Forcemoment ==
  F_T1 : Inport
  F_T2 : Inport  Port=2
  F_T3 : Inport  Port=3
  F_T4 : Inport  Port=4
  F_T5 : Inport  Port=5
  F_T6 : Inport  Port=6
  Constant : Constant  Value=veh.d_T1
  Constant1 : Constant  Value=veh.d_T2
  Constant2 : Constant  Value=veh.d_T3
  Constant3 : Constant  Value=veh.d_T4
  Constant4 : Constant  Value=veh.d_T5
  Constant5 : Constant  Value=veh.d_T6
  Matrix Multiply{,1..5} (6 alike) : Product  Multiplication=Matrix(*)
  m_T1 : Outport
  m_T2 : Outport  Port=2
  m_T3 : Outport  Port=3
  m_T4 : Outport  Port=4
  m_T5 : Outport  Port=5
  m_T6 : Outport  Port=6
  wires:
  F_T2/1 -> Matrix Multiply1/2
  F_T6/1 -> Matrix Multiply5/2
  F_T4/1 -> Matrix Multiply3/2
  Constant/1 -> Matrix Multiply/1
  F_T1/1 -> Matrix Multiply/2
  Constant1/1 -> Matrix Multiply1/1
  Constant2/1 -> Matrix Multiply2/1
  F_T3/1 -> Matrix Multiply2/2
  Constant3/1 -> Matrix Multiply3/1
  Constant4/1 -> Matrix Multiply4/1
  F_T5/1 -> Matrix Multiply4/2
  Constant5/1 -> Matrix Multiply5/1
  Matrix Multiply/1 -> m_T1/1
  Matrix Multiply1/1 -> m_T2/1
  Matrix Multiply2/1 -> m_T3/1
  Matrix Multiply3/1 -> m_T4/1
  Matrix Multiply4/1 -> m_T5/1
  Matrix Multiply5/1 -> m_T6/1

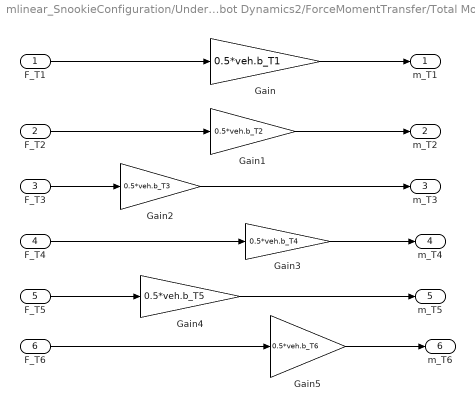
== system mlinear_SnookieConfiguration/Underwater Robot Dynamics2/ForceMomentTransfer/Total Moment/RotationMoment ==
  F_T1 : Inport
  F_T2 : Inport  Port=2
  F_T3 : Inport  Port=3
  F_T4 : Inport  Port=4
  F_T5 : Inport  Port=5
  F_T6 : Inport  Port=6
  Gain : Gain  Gain=0.5*veh.b_T1
  Gain1 : Gain  Gain=0.5*veh.b_T2
  Gain2 : Gain  Gain=0.5*veh.b_T3
  Gain3 : Gain  Gain=0.5*veh.b_T4
  Gain4 : Gain  Gain=0.5*veh.b_T5
  Gain5 : Gain  Gain=0.5*veh.b_T6
  m_T1 : Outport
  m_T2 : Outport  Port=2
  m_T3 : Outport  Port=3
  m_T4 : Outport  Port=4
  m_T5 : Outport  Port=5
  m_T6 : Outport  Port=6
  wires:
  F_T1/1 -> Gain/1
  F_T3/1 -> Gain2/1
  Gain/1 -> m_T1/1
  F_T4/1 -> Gain3/1
  F_T6/1 -> Gain5/1
  F_T2/1 -> Gain1/1
  F_T5/1 -> Gain4/1
  Gain1/1 -> m_T2/1
  Gain2/1 -> m_T3/1
  Gain3/1 -> m_T4/1
  Gain4/1 -> m_T5/1
  Gain5/1 -> m_T6/1

== system mlinear_SnookieConfiguration/Underwater Robot Dynamics2/Underwater Robot Dynamics /6DOF Coriolis forces/3x3 cross product ==
  a : Inport
  b : Inport  Port=2
  Product : Product  SaturateOnIntegerOverflow=on  InputSameDT=on  OutDataTypeStr=Inherit: Same as first input
  Product1 : Product  SaturateOnIntegerOverflow=on  InputSameDT=on  OutDataTypeStr=Inherit: Same as first input
  Selector : Selector  InputPortWidth=3  IndexOptions=Index vector (dialog)  Indices=[2 3 1]  OutputSizes=1
  Selector1 : Selector  InputPortWidth=3  IndexOptions=Index vector (dialog)  Indices=[3 1 2]  OutputSizes=1
  Selector2 : Selector  InputPortWidth=3  IndexOptions=Index vector (dialog)  Indices=[2 3 1]  OutputSizes=1
  Selector3 : Selector  InputPortWidth=3  IndexOptions=Index vector (dialog)  Indices=[3 1 2]  OutputSizes=1
  Sum : Sum  Inputs=+|-  SaturateOnIntegerOverflow=on  InputSameDT=on  OutDataTypeStr=Inherit: Same as first input
  c : Outport  InitialOutput=0
  wires:
  Selector3/1 -> Product1/1
  Selector2/1 -> Product1/2
  Product1/1 -> Sum/2
  Selector1/1 -> Product/2
  Product/1 -> Sum/1
  a/1 -> Selector3/1, Selector/1
  Selector/1 -> Product/1
  b/1 -> Selector2/1, Selector1/1
  Sum/1 -> c/1

== system mlinear_SnookieConfiguration/Underwater Robot Dynamics2/Underwater Robot Dynamics /6DOF Coriolis forces/3x3 cross product 1 ==
  a : Inport
  b : Inport  Port=2
  Product : Product  SaturateOnIntegerOverflow=on  InputSameDT=on  OutDataTypeStr=Inherit: Same as first input
  Product1 : Product  SaturateOnIntegerOverflow=on  InputSameDT=on  OutDataTypeStr=Inherit: Same as first input
  Selector : Selector  InputPortWidth=3  IndexOptions=Index vector (dialog)  Indices=[2 3 1]  OutputSizes=1
  Selector1 : Selector  InputPortWidth=3  IndexOptions=Index vector (dialog)  Indices=[3 1 2]  OutputSizes=1
  Selector2 : Selector  InputPortWidth=3  IndexOptions=Index vector (dialog)  Indices=[2 3 1]  OutputSizes=1
  Selector3 : Selector  InputPortWidth=3  IndexOptions=Index vector (dialog)  Indices=[3 1 2]  OutputSizes=1
  Sum : Sum  Inputs=+|-  SaturateOnIntegerOverflow=on  InputSameDT=on  OutDataTypeStr=Inherit: Same as first input
  c : Outport  InitialOutput=0
  wires:
  Selector3/1 -> Product1/1
  Selector2/1 -> Product1/2
  Product1/1 -> Sum/2
  Selector1/1 -> Product/2
  Product/1 -> Sum/1
  a/1 -> Selector3/1, Selector/1
  Selector/1 -> Product/1
  b/1 -> Selector2/1, Selector1/1
  Sum/1 -> c/1

== system mlinear_SnookieConfiguration/Underwater Robot Dynamics2/Underwater Robot Dynamics /6DOF Coriolis forces/3x3 cross product 2 ==
  a : Inport
  b : Inport  Port=2
  Product : Product  SaturateOnIntegerOverflow=on  InputSameDT=on  OutDataTypeStr=Inherit: Same as first input
  Product1 : Product  SaturateOnIntegerOverflow=on  InputSameDT=on  OutDataTypeStr=Inherit: Same as first input
  Selector : Selector  InputPortWidth=3  IndexOptions=Index vector (dialog)  Indices=[2 3 1]  OutputSizes=1
  Selector1 : Selector  InputPortWidth=3  IndexOptions=Index vector (dialog)  Indices=[3 1 2]  OutputSizes=1
  Selector2 : Selector  InputPortWidth=3  IndexOptions=Index vector (dialog)  Indices=[2 3 1]  OutputSizes=1
  Selector3 : Selector  InputPortWidth=3  IndexOptions=Index vector (dialog)  Indices=[3 1 2]  OutputSizes=1
  Sum : Sum  Inputs=+|-  SaturateOnIntegerOverflow=on  InputSameDT=on  OutDataTypeStr=Inherit: Same as first input
  c : Outport  InitialOutput=0
  wires:
  Selector3/1 -> Product1/1
  Selector2/1 -> Product1/2
  Product1/1 -> Sum/2
  Selector1/1 -> Product/2
  Product/1 -> Sum/1
  a/1 -> Selector3/1, Selector/1
  Selector/1 -> Product/1
  b/1 -> Selector2/1, Selector1/1
  Sum/1 -> c/1
